simulink model "WorkingModel"  (R2020b)
settings: Solver=VariableStepAuto  StartTime=0.0  StopTime=10.0  RelTol=1e-3
model workspace: external: MATLAB File C:\Users\camka\Documents\Code\MATLAB\RiBBIT\Simscape Hexacopter Model\Model_DataFile1.m (data not in the file)
values from neighbouring files (symbols this model uses):
  D = 12    [Startup.m]
  P = 3.8    [Startup.m]
  X = [ 0, 0, 5, 5, 5, 5, 0]*1    [Path_Construction_Demo_Script.m]
  Y = [ 0, 0, 0, 0, 5, 5, 5]*1    [Path_Construction_Demo_Script.m]
  Z = [ 1, 1, 1, 1, 1, 1, 1]*0    [Path_Construction_Demo_Script.m]
undefined symbols (not defined in the file or in its folder): smiData
libraries: sm_lib x705, fl_lib x72, nesl_utility x16
(part 1 of 12)
settings Model: Creator=camka  LastModifiedBy=camka

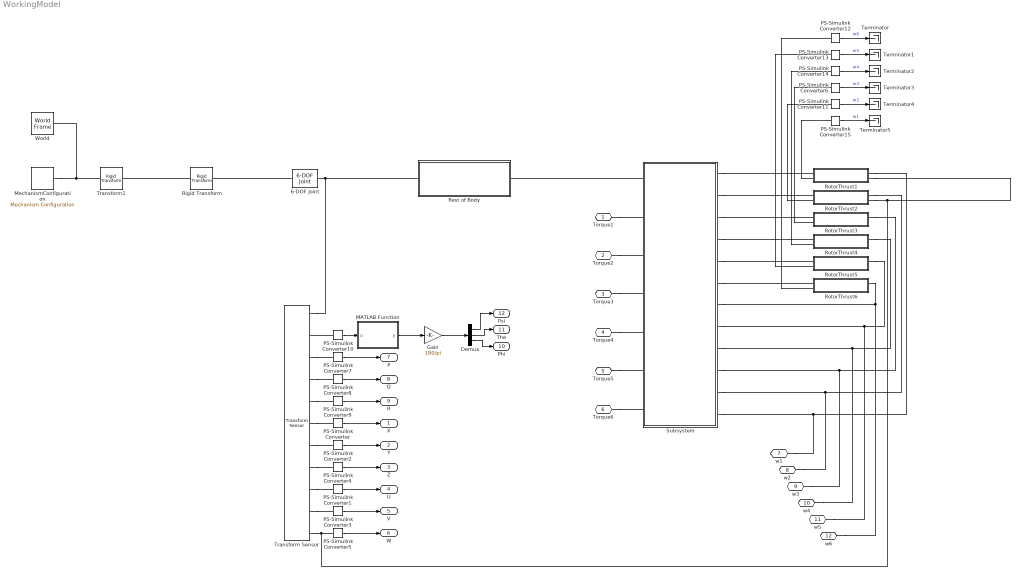
== system WorkingModel ==
  6-DOF Joint : sm_lib/Joints/6-DOF Joint  JointMode=Normal  SenseConstraintForce=off  SenseConstraintForceX=off  SenseConstraintForceY=off  SenseConstraintForceZ=off  SenseConstraintTorque=off  SenseConstraintTorqueX=off  SenseConstraintTorqueY=off  SenseConstraintTorqueZ=off  SenseTotalForce=off  SenseTotalForceX=off  SenseTotalForceY=off  SenseTotalForceZ=off  SenseTotalTorque=off  SenseTotalTorqueX=off  SenseTotalTorqueY=off  SenseTotalTorqueZ=off  CompositeWrenchDir=FollowerOnBase  CompositeWrenchFrame=BaseFrame  PxEquilibriumPosition=0  PxEquilibriumPositionUnits=m  PxSpringStiffness=0  PxSpringStiffnessUnits=N/m  PxDampingCoefficient=0  PxDampingCoefficientUnits=N/(m/s)  PxTorqueActuationMode=NoTorque  PxMotionActuationMode=ComputedMotion  PxSensePosition=off  PxSenseVelocity=off  PxSenseAcceleration=off  PxSenseTorqueForce=off  PxSenseLowerLimitTorqueForce=off  PxSenseUpperLimitTorqueForce=off  PxLowerLimitSpecify=off  PxLowerLimitBound=-1  PxLowerLimitBoundUnits=m  PxLowerLimitStiffness=1e6  PxLowerLimitStiffnessUnits=N/m  PxLowerLimitDamping=1e3  PxLowerLimitDampingUnits=N/(m/s)  PxLowerLimitTransitionRegionWidth=1e-4  PxLowerLimitTransitionRegionWidthUnits=m  PxUpperLimitSpecify=off  PxUpperLimitBound=1  PxUpperLimitBoundUnits=m  PxUpperLimitStiffness=1e6  PxUpperLimitStiffnessUnits=N/m  PxUpperLimitDamping=1e3  PxUpperLimitDampingUnits=N/(m/s)  PxUpperLimitTransitionRegionWidth=1e-4  PxUpperLimitTransitionRegionWidthUnits=m  PxPositionTargetSpecify=off  PxPositionTargetPriority=High  PxPositionTargetValue=0  PxPositionTargetValueUnits=m  PxVelocityTargetSpecify=off  PxVelocityTargetPriority=High  PxVelocityTargetValue=0  PxVelocityTargetValueUnits=m/s  PyEquilibriumPosition=0  PyEquilibriumPositionUnits=m  PySpringStiffness=0  PySpringStiffnessUnits=N/m  PyDampingCoefficient=0  PyDampingCoefficientUnits=N/(m/s)  PyTorqueActuationMode=NoTorque  PyMotionActuationMode=ComputedMotion  PySensePosition=off  PySenseVelocity=off  PySenseAcceleration=off  PySenseTorqueForce=off  PySenseLowerLimitTorqueForce=off  PySenseUpperLimitTorqueForce=off  PyLowerLimitSpecify=off  PyLowerLimitBound=-1  PyLowerLimitBoundUnits=m  PyLowerLimitStiffness=1e6  PyLowerLimitStiffnessUnits=N/m  PyLowerLimitDamping=1e3  PyLowerLimitDampingUnits=N/(m/s)  PyLowerLimitTransitionRegionWidth=1e-4  PyLowerLimitTransitionRegionWidthUnits=m  PyUpperLimitSpecify=off  PyUpperLimitBound=1  PyUpperLimitBoundUnits=m  PyUpperLimitStiffness=1e6  PyUpperLimitStiffnessUnits=N/m  PyUpperLimitDamping=1e3  PyUpperLimitDampingUnits=N/(m/s)  PyUpperLimitTransitionRegionWidth=1e-4  PyUpperLimitTransitionRegionWidthUnits=m  PyPositionTargetSpecify=off  PyPositionTargetPriority=High  PyPositionTargetValue=0  PyPositionTargetValueUnits=m  PyVelocityTargetSpecify=off  PyVelocityTargetPriority=High  PyVelocityTargetValue=0  PyVelocityTargetValueUnits=m/s  PzEquilibriumPosition=0  PzEquilibriumPositionUnits=m  PzSpringStiffness=0  PzSpringStiffnessUnits=N/m  PzDampingCoefficient=0  PzDampingCoefficientUnits=N/(m/s)  PzTorqueActuationMode=NoTorque  PzMotionActuationMode=ComputedMotion  PzSensePosition=off  PzSenseVelocity=off  PzSenseAcceleration=off  PzSenseTorqueForce=off  PzSenseLowerLimitTorqueForce=off  PzSenseUpperLimitTorqueForce=off  PzLowerLimitSpecify=off  PzLowerLimitBound=-1  PzLowerLimitBoundUnits=m  PzLowerLimitStiffness=1e6  PzLowerLimitStiffnessUnits=N/m  PzLowerLimitDamping=1e3  PzLowerLimitDampingUnits=N/(m/s)  PzLowerLimitTransitionRegionWidth=1e-4  PzLowerLimitTransitionRegionWidthUnits=m  PzUpperLimitSpecify=off  PzUpperLimitBound=1  PzUpperLimitBoundUnits=m  PzUpperLimitStiffness=1e6  PzUpperLimitStiffnessUnits=N/m  PzUpperLimitDamping=1e3  PzUpperLimitDampingUnits=N/(m/s)  PzUpperLimitTransitionRegionWidth=1e-4  PzUpperLimitTransitionRegionWidthUnits=m  PzPositionTargetSpecify=off  PzPositionTargetPriority=High  PzPositionTargetValue=-1  PzPositionTargetValueUnits=m  PzVelocityTargetSpecify=off  PzVelocityTargetPriority=High  PzVelocityTargetValue=0  PzVelocityTargetValueUnits=m/s  SphDefPosRotationMethod=None  SphDefPosRotationAngleUnits=deg  SphDefPosRotationStandardAxis=+Z  SphDefPosRotationAngle=0  SphDefPosRotationArbitraryAxis=[0 0 1]  SphDefPosFollAlignAxisA=+X  SphDefPosBaseAlignAxisA=+Y  SphDefPosFollAlignAxisB=+Y  SphDefPosBaseAlignAxisB=+Z  SphDefPosRotationSequenceAxes=FollowerAxes  SphDefPosRotationSequence=XYX  SphDefPosRotationSequenceAngles=[0 0 0]  SphDefPosRotationSequenceAnglesUnits=deg  SphDefPosRotationMatrix=[1 0 0; 0 1 0; 0 0 1]  SphEqPosRotationMethod=None  SphEqPosRotationAngleUnits=deg  SphEqPosRotationStandardAxis=+Z  SphEqPosRotationAngle=0  SphEqPosRotationArbitraryAxis=[0 0 1]  SphEqPosFollAlignAxisA=+X  SphEqPosBaseAlignAxisA=+Y  SphEqPosFollAlignAxisB=+Y  SphEqPosBaseAlignAxisB=+Z  SphEqPosRotationSequenceAxes=FollowerAxes  SphEqPosRotationSequence=XYX  SphEqPosRotationSequenceAngles=[0 0 0]  SphEqPosRotationSequenceAnglesUnits=deg  SphEqPosRotationMatrix=[1 0 0; 0 1 0; 0 0 1]  SphSpringStiffness=0  SphSpringStiffnessUnits=N*m/deg  SphDampingCoefficient=0  SphDampingCoefficientUnits=N*m/(deg/s)  SphActuateTorqueX=off  SphActuateTorqueY=off  SphActuateTorqueZ=off  SphActuateTorque=off  SphTorqueActuationMode=NoTorque  SphMotionActuationMode=ComputedMotion  SphActuationFrame=BaseFrame  SphSensePosition=off  SphSenseVelocityX=off  SphSenseVelocityY=off  SphSenseVelocityZ=off  SphSenseVelocity=off  SphSenseAccelerationX=off  SphSenseAccelerationY=off  SphSenseAccelerationZ=off  SphSenseAcceleration=off  SphSenseTorqueX=off  SphSenseTorqueY=off  SphSenseTorqueZ=off  SphSenseTorqueForce=off  SphSenseLowerLimitTorqueMag=off  SphSenseUpperLimitTorqueMag=off  SphSensingFrame=BaseFrame  SphLowerLimitSpecify=off  SphLowerLimitBound=15  SphLowerLimitBoundUnits=deg  SphLowerLimitStiffness=1e4  SphLowerLimitStiffnessUnits=N*m/deg  SphLowerLimitDamping=10  SphLowerLimitDampingUnits=N*m/(deg/s)  SphLowerLimitTransitionRegionWidth=0.1  SphLowerLimitTransitionRegionWidthUnits=deg  SphUpperLimitSpecify=off  SphUpperLimitBound=45  SphUpperLimitBoundUnits=deg  SphUpperLimitStiffness=1e4  SphUpperLimitStiffnessUnits=N*m/deg  SphUpperLimitDamping=10  SphUpperLimitDampingUnits=N*m/(deg/s)  SphUpperLimitTransitionRegionWidth=0.1  SphUpperLimitTransitionRegionWidthUnits=deg  SphPositionTargetRotationMethod=None  SphPositionTargetRotationAngleUnits=deg  SphPositionTargetRotationStandardAxis=+Z  SphPositionTargetRotationAngle=0  SphPositionTargetRotationArbitraryAxis=[0 0 1]  SphPositionTargetFollAlignAxisA=+X  SphPositionTargetBaseAlignAxisA=+Y  SphPositionTargetFollAlignAxisB=+Y  SphPositionTargetBaseAlignAxisB=+Z  SphPositionTargetRotationSequenceAxes=FollowerAxes  SphPositionTargetRotationSequence=XYX  SphPositionTargetRotationSequenceAngles=[0 0 0]  SphPositionTargetRotationSequenceAnglesUnits=deg  SphPositionTargetRotationMatrix=[1 0 0; 0 1 0; 0 0 1]  SphPositionTargetSpecify=off  SphPositionTargetPriority=High  SphVelocityTargetValue=[0 0 0]  SphVelocityTargetValueUnits=deg/s  SphVelocityTargetSpecify=off  SphVelocityTargetPriority=High  SphVelocityTargetInFollowerFrame=on
  Demux : Demux  Outputs=3
  Gain : Gain  Gain=180/pi
  MATLAB Function : MATLAB Function  TreatAsAtomicUnit=on
  MechanismConfiguration : sm_lib/Utilities/Mechanism Configuration  UniformGravity=Constant  GravityVector=[0 0 0]  GravityVectorUnits=m/s^2  GravityUnits=m/s^2  LinearizationDelta=0.001  JointModeTransitionNonlinearIterations=2
  PS-Simulink Converter{,1..15} (16 alike) : nesl_utility/PS-Simulink Converter  PhysicalDomain=network_engine_domain  SubClassName=ps_output  LeftPortType=input  RightPortType=output  PseudoPeriodic=off  Frequencies=[]  Unit=inherit  AffineConversion=off
  Rest of Body : Subsystem
  Rigid Transform : sm_lib/Frames and Transforms/Rigid Transform  TranslationMethod=None  TranslationStandardOffset=0  TranslationLengthUnit=m  TranslationStandardAxis=+Z  TranslationCartesianOffset=[0 0 0]  TranslationROffset=0  TranslationROffsetUnits=m  TranslationZOffset=0  TranslationZOffsetUnits=m  TranslationThetaOffset=0  TranslationThetaOffsetUnits=deg  RotationMethod=RotationSequence  RotationAngleUnits=deg  RotationStandardAxis=+Z  RotationAngle=0.0  RotationArbitraryAxis=[0 0 1]  FollAlignAxisA=+X  BaseAlignAxisA=+Y  FollAlignAxisB=+Y  BaseAlignAxisB=+Z  RotationSequenceAxes=BaseAxes  RotationSequence=XZX  RotationSequenceAngles=[-90 90 0]  RotationSequenceAnglesUnits=deg  RotationMatrix=[1 0 0; 0 1 0; 0 0 1]
  RotorThrust1 : Subsystem
  RotorThrust2 : Subsystem
  RotorThrust3 : Subsystem
  RotorThrust4 : Subsystem
  RotorThrust5 : Subsystem
  RotorThrust6 : Subsystem
  Subsystem : Subsystem
  Terminator{,1..5} (6 alike) : Terminator
  Transform Sensor : sm_lib/Frames and Transforms/Transform Sensor  MeasurementFrame=NonRotatingBase  SenseAngle=off  SenseAxis=off  SenseAngle1=off  SenseAngle2=off  SenseAngle3=off  SenseQ=on  SenseR=off  SenseOmegaX=on  SenseOmegaY=on  SenseOmegaZ=on  SenseOmega1=off  SenseOmega2=off  SenseOmega3=off  SenseQDot=off  SenseRDot=off  SenseAlphaX=off  SenseAlphaY=off  SenseAlphaZ=off  SenseAlpha1=off  SenseAlpha2=off  SenseAlpha3=off  SenseQDDot=off  SenseRDDot=off  SenseX=on  SenseY=on  SenseZ=on  SenseRad=off  SenseAzim=off  SenseDist=off  SenseInc=off  SenseXDot=on  SenseYDot=on  SenseZDot=on  SenseRadDot=off  SenseAzimDot=off  SenseDistDot=off  SenseIncDot=off  SenseXDDot=off  SenseYDDot=off  SenseZDDot=off  SenseRadDDot=off  SenseAzimDDot=off  SenseDistDDot=off  SenseIncDDot=off
  Transform1 : sm_lib/Frames and Transforms/Rigid Transform  TranslationMethod=Cartesian  TranslationStandardOffset=0  TranslationLengthUnit=cm  TranslationStandardAxis=+Z  TranslationCartesianOffset=smiData.RigidTransform(6).translation  TranslationROffset=0  TranslationROffsetUnits=m  TranslationZOffset=0  TranslationZOffsetUnits=m  TranslationThetaOffset=0  TranslationThetaOffsetUnits=deg  RotationMethod=ArbitraryAxis  RotationAngleUnits=rad  RotationStandardAxis=+Z  RotationAngle=smiData.RigidTransform(6).angle  RotationArbitraryAxis=smiData.RigidTransform(6).axis  FollAlignAxisA=+X  BaseAlignAxisA=+Y  FollAlignAxisB=+Y  BaseAlignAxisB=+Z  RotationSequenceAxes=FollowerAxes  RotationSequence=XYX  RotationSequenceAngles=[0 0 0]  RotationSequenceAnglesUnits=deg  RotationMatrix=[1 0 0; 0 1 0; 0 0 1]
  World : sm_lib/Frames and Transforms/World Frame
  Torque1 : PMIOPort  Side=Left
  Torque2 : PMIOPort  Port=2  Side=Left
  Torque3 : PMIOPort  Port=3  Side=Left
  Torque4 : PMIOPort  Port=4  Side=Left
  Torque5 : PMIOPort  Port=5  Side=Left
  Torque6 : PMIOPort  Port=6  Side=Left
  w1 : PMIOPort  Port=7  Side=Left
  w2 : PMIOPort  Port=8  Side=Left
  w3 : PMIOPort  Port=9  Side=Left
  w4 : PMIOPort  Port=10  Side=Left
  w5 : PMIOPort  Port=11  Side=Left
  w6 : PMIOPort  Port=12  Side=Left
  X : Outport
  Y : Outport  Port=2
  Z : Outport  Port=3
  U : Outport  Port=4
  V : Outport  Port=5
  W : Outport  Port=6
  P : Outport  Port=7
  Q : Outport  Port=8
  R : Outport  Port=9
  Phi : Outport  Port=10
  The : Outport  Port=11
  Psi : Outport  Port=12
  wires:
  Demux/2 -> The/1
  PS-Simulink Converter10/1 -> MATLAB Function/1(u)
  MATLAB Function/1(y) -> Gain/1
  PS-Simulink Converter1/1 -> U/1
  PS-Simulink Converter/1 -> X/1
  Demux/3 -> Phi/1
  PS-Simulink Converter4/1 -> Z/1
  PS-Simulink Converter3/1 -> V/1
  Demux/1 -> Psi/1
  PS-Simulink Converter7/1 -> P/1
  PS-Simulink Converter5/1 -> W/1
  PS-Simulink Converter8/1 -> Q/1
  PS-Simulink Converter2/1 -> Y/1
  PS-Simulink Converter9/1 -> R/1
  Gain/1 -> Demux/1
  PS-Simulink Converter13/1 -> Terminator1/1  "w5"
  PS-Simulink Converter14/1 -> Terminator2/1  "w4"
  PS-Simulink Converter12/1 -> Terminator/1  "w6"
  PS-Simulink Converter6/1 -> Terminator3/1  "w3"
  PS-Simulink Converter11/1 -> Terminator4/1  "w2"
  PS-Simulink Converter15/1 -> Terminator5/1  "w1"
  connections:
  World/RConn1 -- MechanismConfiguration/RConn1 -- Transform1/LConn1
  Rigid Transform/LConn1 -- Transform1/RConn1
  RotorThrust2/LConn2 -- RotorThrust1/LConn2 -- Transform Sensor/RConn11 -- PS-Simulink Converter5/LConn1
  Transform Sensor/RConn4 -- PS-Simulink Converter8/LConn1
  Transform Sensor/RConn9 -- PS-Simulink Converter1/LConn1
  Transform Sensor/RConn7 -- PS-Simulink Converter2/LConn1
  Transform Sensor/RConn8 -- PS-Simulink Converter4/LConn1
  6-DOF Joint/RConn1 -- Rest of Body/RConn1 -- Transform Sensor/RConn1
  Transform Sensor/RConn6 -- PS-Simulink Converter/LConn1
  Transform Sensor/RConn3 -- PS-Simulink Converter7/LConn1
  6-DOF Joint/LConn1 -- Rigid Transform/RConn1
  Transform Sensor/RConn10 -- PS-Simulink Converter3/LConn1
  Transform Sensor/RConn5 -- PS-Simulink Converter9/LConn1
  PS-Simulink Converter10/LConn1 -- Transform Sensor/RConn2
  Subsystem/LConn1 -- Rest of Body/LConn1
  RotorThrust4/LConn1 -- Subsystem/RConn9 -- w4/RConn1
  RotorThrust3/LConn1 -- Subsystem/RConn10 -- w3/RConn1
  RotorThrust2/LConn1 -- Subsystem/RConn11 -- w2/RConn1
  RotorThrust6/LConn1 -- Subsystem/RConn7 -- w6/RConn1
  RotorThrust5/LConn1 -- Subsystem/RConn8 -- w5/RConn1
  RotorThrust1/LConn1 -- Subsystem/RConn12 -- w1/RConn1
  PS-Simulink Converter12/LConn1 -- RotorThrust6/RConn2
  Subsystem/RConn6 -- RotorThrust6/RConn1
  Subsystem/RConn2 -- RotorThrust2/RConn1
  PS-Simulink Converter11/LConn1 -- RotorThrust2/RConn2
  PS-Simulink Converter6/LConn1 -- RotorThrust3/RConn2
  PS-Simulink Converter15/LConn1 -- RotorThrust1/RConn2
  PS-Simulink Converter13/LConn1 -- RotorThrust5/RConn2
  PS-Simulink Converter14/LConn1 -- RotorThrust4/RConn2
  Subsystem/RConn5 -- RotorThrust5/RConn1
  Subsystem/RConn3 -- RotorThrust3/RConn1
  Subsystem/RConn4 -- RotorThrust4/RConn1
  Subsystem/RConn1 -- RotorThrust1/RConn1
  Torque1/RConn1 -- Subsystem/LConn2
  Torque2/RConn1 -- Subsystem/LConn3
  Torque3/RConn1 -- Subsystem/LConn4
  Torque4/RConn1 -- Subsystem/LConn5
  Torque5/RConn1 -- Subsystem/LConn6
  Torque6/RConn1 -- Subsystem/LConn7

== system WorkingModel/Rest of Body ==
  ReferenceFrame : sm_lib/Frames and Transforms/Reference Frame
  ReferenceFrame1 : sm_lib/Frames and Transforms/Reference Frame
  ReferenceFrame2 : sm_lib/Frames and Transforms/Reference Frame
  Subsystem : Subsystem
  Subsystem1 : Subsystem
  Transform1 : sm_lib/Frames and Transforms/Rigid Transform  TranslationMethod=Cartesian  TranslationStandardOffset=0  TranslationLengthUnit=cm  TranslationStandardAxis=+Z  TranslationCartesianOffset=smiData.RigidTransform(5).translation  TranslationROffset=0  TranslationROffsetUnits=m  TranslationZOffset=0  TranslationZOffsetUnits=m  TranslationThetaOffset=0  TranslationThetaOffsetUnits=deg  RotationMethod=ArbitraryAxis  RotationAngleUnits=rad  RotationStandardAxis=+Z  RotationAngle=smiData.RigidTransform(5).angle  RotationArbitraryAxis=smiData.RigidTransform(5).axis  FollAlignAxisA=+X  BaseAlignAxisA=+Y  FollAlignAxisB=+Y  BaseAlignAxisB=+Z  RotationSequenceAxes=FollowerAxes  RotationSequence=XYX  RotationSequenceAngles=[0 0 0]  RotationSequenceAnglesUnits=deg  RotationMatrix=[1 0 0; 0 1 0; 0 0 1]
  Transform34 : sm_lib/Frames and Transforms/Rigid Transform  TranslationMethod=Cartesian  TranslationStandardOffset=0  TranslationLengthUnit=cm  TranslationStandardAxis=+Z  TranslationCartesianOffset=smiData.RigidTransform(128).translation  TranslationROffset=0  TranslationROffsetUnits=m  TranslationZOffset=0  TranslationZOffsetUnits=m  TranslationThetaOffset=0  TranslationThetaOffsetUnits=deg  RotationMethod=ArbitraryAxis  RotationAngleUnits=rad  RotationStandardAxis=+Z  RotationAngle=smiData.RigidTransform(128).angle  RotationArbitraryAxis=smiData.RigidTransform(128).axis  FollAlignAxisA=+X  BaseAlignAxisA=+Y  FollAlignAxisB=+Y  BaseAlignAxisB=+Z  RotationSequenceAxes=FollowerAxes  RotationSequence=XYX  RotationSequenceAngles=[0 0 0]  RotationSequenceAnglesUnits=deg  RotationMatrix=[1 0 0; 0 1 0; 0 0 1]
  Transform5 : sm_lib/Frames and Transforms/Rigid Transform  TranslationMethod=Cartesian  TranslationStandardOffset=0  TranslationLengthUnit=cm  TranslationStandardAxis=+Z  TranslationCartesianOffset=smiData.RigidTransform(236).translation  TranslationROffset=0  TranslationROffsetUnits=m  TranslationZOffset=0  TranslationZOffsetUnits=m  TranslationThetaOffset=0  TranslationThetaOffsetUnits=deg  RotationMethod=ArbitraryAxis  RotationAngleUnits=rad  RotationStandardAxis=+Z  RotationAngle=smiData.RigidTransform(236).angle  RotationArbitraryAxis=smiData.RigidTransform(236).axis  FollAlignAxisA=+X  BaseAlignAxisA=+Y  FollAlignAxisB=+Y  BaseAlignAxisB=+Z  RotationSequenceAxes=FollowerAxes  RotationSequence=XYX  RotationSequenceAngles=[0 0 0]  RotationSequenceAnglesUnits=deg  RotationMatrix=[1 0 0; 0 1 0; 0 0 1]
  Transform2 : PMIOPort  Side=Right
  Transform3 : PMIOPort  Port=2  Side=Left
  connections:
  Transform1/LConn1 -- Transform5/LConn1 -- ReferenceFrame/RConn1
  ReferenceFrame1/RConn1 -- Transform3/RConn1 -- Transform34/RConn1 -- Subsystem1/LConn1
  ReferenceFrame2/RConn1 -- Transform34/LConn1 -- Subsystem/LConn1 -- Transform5/RConn1
  Transform1/RConn1 -- Transform2/RConn1

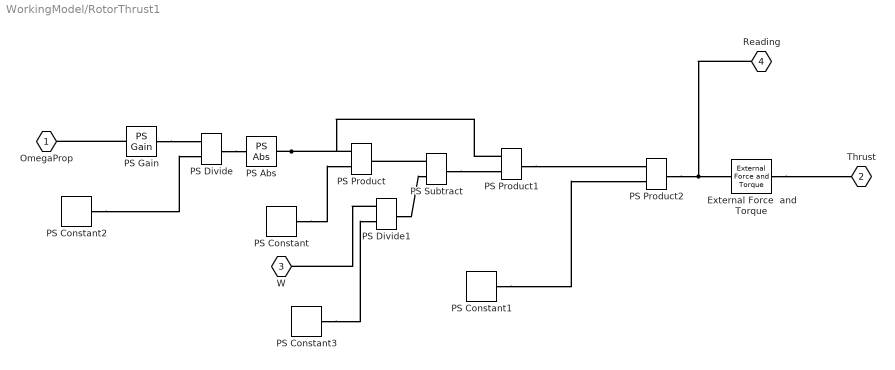
== system WorkingModel/RotorThrust1 ==
  External Force  and Torque : sm_lib/Forces and Torques/External Force and Torque  ForceResolutionFrame=AttachedFrame  EnableForceX=off  EnableForceY=off  EnableForceZ=on  EnableForce=off  TorqueResolutionFrame=AttachedFrame  EnableTorqueX=off  EnableTorqueY=off  EnableTorqueZ=off  EnableTorque=off
  PS Abs : fl_lib/Physical Signals/Nonlinear Operators/PS Abs
      settings: SourceProductBaseCode=SS  InternalSimscapePortConfiguration="{\"Bottom\":[],\"Left\":[{\"id\":\"I\",\"label\":\"\",\"type\":\"input\"}],\"Right\":[{\"id\":\"O\",\"label\":\"\",\"type\":\"output\"}],\"Top\":[]}"
  PS Constant : fl_lib/Physical Signals/Sources/PS Constant  constant=4.23333e-4*P
  PS Constant1 : fl_lib/Physical Signals/Sources/PS Constant  constant=4.392399e-8*D^3.5/sqrt(P) N
  PS Constant2 : fl_lib/Physical Signals/Sources/PS Constant  constant=1 rad/s
  PS Constant3 : fl_lib/Physical Signals/Sources/PS Constant  constant=1 m/s
  PS Divide : fl_lib/Physical Signals/Functions/PS Divide
      settings: SourceProductBaseCode=SS
  PS Divide1 : fl_lib/Physical Signals/Functions/PS Divide
      settings: SourceProductBaseCode=SS
  PS Gain : fl_lib/Physical Signals/Functions/PS Gain  gain=30/pi
  PS Product : fl_lib/Physical Signals/Functions/PS Product
  PS Product1 : fl_lib/Physical Signals/Functions/PS Product
  PS Product2 : fl_lib/Physical Signals/Functions/PS Product
  PS Subtract : fl_lib/Physical Signals/Functions/PS Subtract
  OmegaProp : PMIOPort  Side=Left
  Thrust : PMIOPort  Port=2  Side=Right
  W : PMIOPort  Port=3  Side=Left
  Reading : PMIOPort  Port=4  Side=Right
  connections:
  External Force  and Torque/RConn1 -- Thrust/RConn1
  PS Product2/RConn1 -- Reading/RConn1 -- External Force  and Torque/LConn1
  PS Gain/LConn1 -- OmegaProp/RConn1
  PS Constant/RConn1 -- PS Product/LConn2
  PS Abs/RConn1 -- PS Product/LConn1 -- PS Product1/LConn1
  PS Subtract/LConn1 -- PS Product/RConn1
  PS Divide1/LConn1 -- W/RConn1
  PS Subtract/RConn1 -- PS Product1/LConn2
  PS Constant1/RConn1 -- PS Product2/LConn2
  PS Product1/RConn1 -- PS Product2/LConn1
  PS Gain/RConn1 -- PS Divide/LConn1
  PS Divide/RConn1 -- PS Abs/LConn1
  PS Constant2/RConn1 -- PS Divide/LConn2
  PS Divide1/RConn1 -- PS Subtract/LConn2
  PS Constant3/RConn1 -- PS Divide1/LConn2

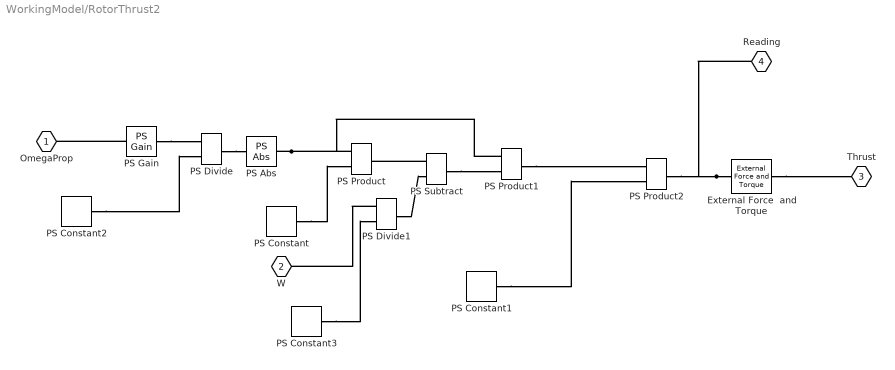
== system WorkingModel/RotorThrust2 ==
  External Force  and Torque : sm_lib/Forces and Torques/External Force and Torque  ForceResolutionFrame=AttachedFrame  EnableForceX=off  EnableForceY=off  EnableForceZ=on  EnableForce=off  TorqueResolutionFrame=AttachedFrame  EnableTorqueX=off  EnableTorqueY=off  EnableTorqueZ=off  EnableTorque=off
  PS Abs : fl_lib/Physical Signals/Nonlinear Operators/PS Abs
      settings: SourceProductBaseCode=SS  InternalSimscapePortConfiguration="{\"Bottom\":[],\"Left\":[{\"id\":\"I\",\"label\":\"\",\"type\":\"input\"}],\"Right\":[{\"id\":\"O\",\"label\":\"\",\"type\":\"output\"}],\"Top\":[]}"
  PS Constant : fl_lib/Physical Signals/Sources/PS Constant  constant=4.23333e-4*P
  PS Constant1 : fl_lib/Physical Signals/Sources/PS Constant  constant=4.392399e-8*D^3.5/sqrt(P) N
  PS Constant2 : fl_lib/Physical Signals/Sources/PS Constant  constant=1 rad/s
  PS Constant3 : fl_lib/Physical Signals/Sources/PS Constant  constant=1 m/s
  PS Divide : fl_lib/Physical Signals/Functions/PS Divide
      settings: SourceProductBaseCode=SS
  PS Divide1 : fl_lib/Physical Signals/Functions/PS Divide
      settings: SourceProductBaseCode=SS
  PS Gain : fl_lib/Physical Signals/Functions/PS Gain  gain=30/pi
  PS Product : fl_lib/Physical Signals/Functions/PS Product
  PS Product1 : fl_lib/Physical Signals/Functions/PS Product
  PS Product2 : fl_lib/Physical Signals/Functions/PS Product
  PS Subtract : fl_lib/Physical Signals/Functions/PS Subtract
  OmegaProp : PMIOPort  Side=Left
  W : PMIOPort  Port=2  Side=Left
  Thrust : PMIOPort  Port=3  Side=Right
  Reading : PMIOPort  Port=4  Side=Right
  connections:
  External Force  and Torque/RConn1 -- Thrust/RConn1
  External Force  and Torque/LConn1 -- PS Product2/RConn1 -- Reading/RConn1
  PS Gain/LConn1 -- OmegaProp/RConn1
  PS Constant/RConn1 -- PS Product/LConn2
  PS Abs/RConn1 -- PS Product/LConn1 -- PS Product1/LConn1
  PS Subtract/LConn1 -- PS Product/RConn1
  PS Divide1/LConn1 -- W/RConn1
  PS Subtract/RConn1 -- PS Product1/LConn2
  PS Constant1/RConn1 -- PS Product2/LConn2
  PS Product1/RConn1 -- PS Product2/LConn1
  PS Gain/RConn1 -- PS Divide/LConn1
  PS Divide/RConn1 -- PS Abs/LConn1
  PS Constant2/RConn1 -- PS Divide/LConn2
  PS Divide1/RConn1 -- PS Subtract/LConn2
  PS Constant3/RConn1 -- PS Divide1/LConn2

== system WorkingModel/RotorThrust3 ==
  External Force  and Torque : sm_lib/Forces and Torques/External Force and Torque  ForceResolutionFrame=AttachedFrame  EnableForceX=off  EnableForceY=off  EnableForceZ=on  EnableForce=off  TorqueResolutionFrame=AttachedFrame  EnableTorqueX=off  EnableTorqueY=off  EnableTorqueZ=off  EnableTorque=off
  PS Abs : fl_lib/Physical Signals/Nonlinear Operators/PS Abs
      settings: SourceProductBaseCode=SS  InternalSimscapePortConfiguration="{\"Bottom\":[],\"Left\":[{\"id\":\"I\",\"label\":\"\",\"type\":\"input\"}],\"Right\":[{\"id\":\"O\",\"label\":\"\",\"type\":\"output\"}],\"Top\":[]}"
  PS Constant : fl_lib/Physical Signals/Sources/PS Constant  constant=4.23333e-4*P
  PS Constant1 : fl_lib/Physical Signals/Sources/PS Constant  constant=4.392399e-8*D^3.5/sqrt(P) N
  PS Constant2 : fl_lib/Physical Signals/Sources/PS Constant  constant=1 rad/s
  PS Constant3 : fl_lib/Physical Signals/Sources/PS Constant  constant=1 m/s
  PS Divide : fl_lib/Physical Signals/Functions/PS Divide
      settings: SourceProductBaseCode=SS
  PS Divide1 : fl_lib/Physical Signals/Functions/PS Divide
      settings: SourceProductBaseCode=SS
  PS Gain : fl_lib/Physical Signals/Functions/PS Gain  gain=30/pi
  PS Product : fl_lib/Physical Signals/Functions/PS Product
  PS Product1 : fl_lib/Physical Signals/Functions/PS Product
  PS Product2 : fl_lib/Physical Signals/Functions/PS Product
  PS Subtract : fl_lib/Physical Signals/Functions/PS Subtract
  OmegaProp : PMIOPort  Side=Left
  Thrust : PMIOPort  Port=2  Side=Right
  W : PMIOPort  Port=3  Side=Left
  Reading : PMIOPort  Port=4  Side=Right
  connections:
  External Force  and Torque/RConn1 -- Thrust/RConn1
  External Force  and Torque/LConn1 -- PS Product2/RConn1 -- Reading/RConn1
  PS Gain/LConn1 -- OmegaProp/RConn1
  PS Constant/RConn1 -- PS Product/LConn2
  PS Abs/RConn1 -- PS Product/LConn1 -- PS Product1/LConn1
  PS Subtract/LConn1 -- PS Product/RConn1
  PS Divide1/LConn1 -- W/RConn1
  PS Subtract/RConn1 -- PS Product1/LConn2
  PS Constant1/RConn1 -- PS Product2/LConn2
  PS Product1/RConn1 -- PS Product2/LConn1
  PS Gain/RConn1 -- PS Divide/LConn1
  PS Divide/RConn1 -- PS Abs/LConn1
  PS Constant2/RConn1 -- PS Divide/LConn2
  PS Divide1/RConn1 -- PS Subtract/LConn2
  PS Constant3/RConn1 -- PS Divide1/LConn2

== system WorkingModel/RotorThrust4 ==
  External Force  and Torque : sm_lib/Forces and Torques/External Force and Torque  ForceResolutionFrame=AttachedFrame  EnableForceX=off  EnableForceY=off  EnableForceZ=on  EnableForce=off  TorqueResolutionFrame=AttachedFrame  EnableTorqueX=off  EnableTorqueY=off  EnableTorqueZ=off  EnableTorque=off
  PS Abs : fl_lib/Physical Signals/Nonlinear Operators/PS Abs
      settings: SourceProductBaseCode=SS  InternalSimscapePortConfiguration="{\"Bottom\":[],\"Left\":[{\"id\":\"I\",\"label\":\"\",\"type\":\"input\"}],\"Right\":[{\"id\":\"O\",\"label\":\"\",\"type\":\"output\"}],\"Top\":[]}"
  PS Constant : fl_lib/Physical Signals/Sources/PS Constant  constant=4.23333e-4*P
  PS Constant1 : fl_lib/Physical Signals/Sources/PS Constant  constant=4.392399e-8*D^3.5/sqrt(P) N
  PS Constant2 : fl_lib/Physical Signals/Sources/PS Constant  constant=1 rad/s
  PS Constant3 : fl_lib/Physical Signals/Sources/PS Constant  constant=1 m/s
  PS Divide : fl_lib/Physical Signals/Functions/PS Divide
      settings: SourceProductBaseCode=SS
  PS Divide1 : fl_lib/Physical Signals/Functions/PS Divide
      settings: SourceProductBaseCode=SS
  PS Gain : fl_lib/Physical Signals/Functions/PS Gain  gain=30/pi
  PS Product : fl_lib/Physical Signals/Functions/PS Product
  PS Product1 : fl_lib/Physical Signals/Functions/PS Product
  PS Product2 : fl_lib/Physical Signals/Functions/PS Product
  PS Subtract : fl_lib/Physical Signals/Functions/PS Subtract
  OmegaProp : PMIOPort  Side=Left
  Thrust : PMIOPort  Port=2  Side=Right
  W : PMIOPort  Port=3  Side=Left
  Reading : PMIOPort  Port=4  Side=Right
  connections:
  External Force  and Torque/RConn1 -- Thrust/RConn1
  External Force  and Torque/LConn1 -- PS Product2/RConn1 -- Reading/RConn1
  PS Gain/LConn1 -- OmegaProp/RConn1
  PS Constant/RConn1 -- PS Product/LConn2
  PS Abs/RConn1 -- PS Product/LConn1 -- PS Product1/LConn1
  PS Subtract/LConn1 -- PS Product/RConn1
  PS Divide1/LConn1 -- W/RConn1
  PS Subtract/RConn1 -- PS Product1/LConn2
  PS Constant1/RConn1 -- PS Product2/LConn2
  PS Product1/RConn1 -- PS Product2/LConn1
  PS Gain/RConn1 -- PS Divide/LConn1
  PS Divide/RConn1 -- PS Abs/LConn1
  PS Constant2/RConn1 -- PS Divide/LConn2
  PS Divide1/RConn1 -- PS Subtract/LConn2
  PS Constant3/RConn1 -- PS Divide1/LConn2

== system WorkingModel/RotorThrust5 ==
  External Force  and Torque : sm_lib/Forces and Torques/External Force and Torque  ForceResolutionFrame=AttachedFrame  EnableForceX=off  EnableForceY=off  EnableForceZ=on  EnableForce=off  TorqueResolutionFrame=AttachedFrame  EnableTorqueX=off  EnableTorqueY=off  EnableTorqueZ=off  EnableTorque=off
  PS Abs : fl_lib/Physical Signals/Nonlinear Operators/PS Abs
      settings: SourceProductBaseCode=SS  InternalSimscapePortConfiguration="{\"Bottom\":[],\"Left\":[{\"id\":\"I\",\"label\":\"\",\"type\":\"input\"}],\"Right\":[{\"id\":\"O\",\"label\":\"\",\"type\":\"output\"}],\"Top\":[]}"
  PS Constant : fl_lib/Physical Signals/Sources/PS Constant  constant=4.23333e-4*P
  PS Constant1 : fl_lib/Physical Signals/Sources/PS Constant  constant=4.392399e-8*D^3.5/sqrt(P) N
  PS Constant2 : fl_lib/Physical Signals/Sources/PS Constant  constant=1 rad/s
  PS Constant3 : fl_lib/Physical Signals/Sources/PS Constant  constant=1 m/s
  PS Divide : fl_lib/Physical Signals/Functions/PS Divide
      settings: SourceProductBaseCode=SS
  PS Divide1 : fl_lib/Physical Signals/Functions/PS Divide
      settings: SourceProductBaseCode=SS
  PS Gain : fl_lib/Physical Signals/Functions/PS Gain  gain=30/pi
  PS Product : fl_lib/Physical Signals/Functions/PS Product
  PS Product1 : fl_lib/Physical Signals/Functions/PS Product
  PS Product2 : fl_lib/Physical Signals/Functions/PS Product
  PS Subtract : fl_lib/Physical Signals/Functions/PS Subtract
  OmegaProp : PMIOPort  Side=Left
  Thrust : PMIOPort  Port=2  Side=Right
  W : PMIOPort  Port=3  Side=Left
  Reading : PMIOPort  Port=4  Side=Right
  connections:
  External Force  and Torque/RConn1 -- Thrust/RConn1
  External Force  and Torque/LConn1 -- PS Product2/RConn1 -- Reading/RConn1
  PS Gain/LConn1 -- OmegaProp/RConn1
  PS Constant/RConn1 -- PS Product/LConn2
  PS Abs/RConn1 -- PS Product/LConn1 -- PS Product1/LConn1
  PS Subtract/LConn1 -- PS Product/RConn1
  PS Divide1/LConn1 -- W/RConn1
  PS Subtract/RConn1 -- PS Product1/LConn2
  PS Constant1/RConn1 -- PS Product2/LConn2
  PS Product1/RConn1 -- PS Product2/LConn1
  PS Gain/RConn1 -- PS Divide/LConn1
  PS Divide/RConn1 -- PS Abs/LConn1
  PS Constant2/RConn1 -- PS Divide/LConn2
  PS Divide1/RConn1 -- PS Subtract/LConn2
  PS Constant3/RConn1 -- PS Divide1/LConn2

== system WorkingModel/RotorThrust6 ==
  External Force  and Torque : sm_lib/Forces and Torques/External Force and Torque  ForceResolutionFrame=AttachedFrame  EnableForceX=off  EnableForceY=off  EnableForceZ=on  EnableForce=off  TorqueResolutionFrame=AttachedFrame  EnableTorqueX=off  EnableTorqueY=off  EnableTorqueZ=off  EnableTorque=off
  PS Abs : fl_lib/Physical Signals/Nonlinear Operators/PS Abs
      settings: SourceProductBaseCode=SS  InternalSimscapePortConfiguration="{\"Bottom\":[],\"Left\":[{\"id\":\"I\",\"label\":\"\",\"type\":\"input\"}],\"Right\":[{\"id\":\"O\",\"label\":\"\",\"type\":\"output\"}],\"Top\":[]}"
  PS Constant : fl_lib/Physical Signals/Sources/PS Constant  constant=4.23333e-4*P
  PS Constant1 : fl_lib/Physical Signals/Sources/PS Constant  constant=4.392399e-8*D^3.5/sqrt(P) N
  PS Constant2 : fl_lib/Physical Signals/Sources/PS Constant  constant=1 rad/s
  PS Constant3 : fl_lib/Physical Signals/Sources/PS Constant  constant=1 m/s
  PS Divide : fl_lib/Physical Signals/Functions/PS Divide
      settings: SourceProductBaseCode=SS
  PS Divide1 : fl_lib/Physical Signals/Functions/PS Divide
      settings: SourceProductBaseCode=SS
  PS Gain : fl_lib/Physical Signals/Functions/PS Gain  gain=30/pi
  PS Product : fl_lib/Physical Signals/Functions/PS Product
  PS Product1 : fl_lib/Physical Signals/Functions/PS Product
  PS Product2 : fl_lib/Physical Signals/Functions/PS Product
  PS Subtract : fl_lib/Physical Signals/Functions/PS Subtract
  OmegaProp : PMIOPort  Side=Left
  Thrust : PMIOPort  Port=2  Side=Right
  W : PMIOPort  Port=3  Side=Left
  Reading : PMIOPort  Port=4  Side=Right
  connections:
  External Force  and Torque/RConn1 -- Thrust/RConn1
  External Force  and Torque/LConn1 -- PS Product2/RConn1 -- Reading/RConn1
  PS Gain/LConn1 -- OmegaProp/RConn1
  PS Constant/RConn1 -- PS Product/LConn2
  PS Abs/RConn1 -- PS Product/LConn1 -- PS Product1/LConn1
  PS Subtract/LConn1 -- PS Product/RConn1
  PS Divide1/LConn1 -- W/RConn1
  PS Subtract/RConn1 -- PS Product1/LConn2
  PS Constant1/RConn1 -- PS Product2/LConn2
  PS Product1/RConn1 -- PS Product2/LConn1
  PS Gain/RConn1 -- PS Divide/LConn1
  PS Divide/RConn1 -- PS Abs/LConn1
  PS Constant2/RConn1 -- PS Divide/LConn2
  PS Divide1/RConn1 -- PS Subtract/LConn2
  PS Constant3/RConn1 -- PS Divide1/LConn2

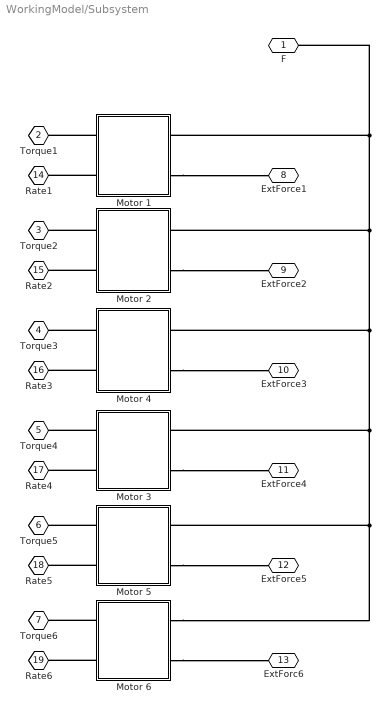
== system WorkingModel/Subsystem ==
  Motor 1 : Subsystem
  Motor 2 : Subsystem
  Motor 3 : Subsystem
  Motor 4 : Subsystem
  Motor 5 : Subsystem
  Motor 6 : Subsystem
  F : PMIOPort  Side=Left
  Torque1 : PMIOPort  Tag=PMCPort  Port=2  Side=Left
  Torque2 : PMIOPort  Tag=PMCPort  Port=3  Side=Left
  Torque3 : PMIOPort  Tag=PMCPort  Port=4  Side=Left
  Torque4 : PMIOPort  Tag=PMCPort  Port=5  Side=Left
  Torque5 : PMIOPort  Tag=PMCPort  Port=6  Side=Left
  Torque6 : PMIOPort  Tag=PMCPort  Port=7  Side=Left
  ExtForce1 : PMIOPort  Port=8  Side=Right
  ExtForce2 : PMIOPort  Port=9  Side=Right
  ExtForce3 : PMIOPort  Port=10  Side=Right
  ExtForce4 : PMIOPort  Port=11  Side=Right
  ExtForce5 : PMIOPort  Port=12  Side=Right
  ExtForc6 : PMIOPort  Port=13  Side=Right
  Rate1 : PMIOPort  Tag=PMCPort  Port=14  Side=Right
  Rate2 : PMIOPort  Tag=PMCPort  Port=15  Side=Right
  Rate3 : PMIOPort  Tag=PMCPort  Port=16  Side=Right
  Rate4 : PMIOPort  Tag=PMCPort  Port=17  Side=Right
  Rate5 : PMIOPort  Tag=PMCPort  Port=18  Side=Right
  Rate6 : PMIOPort  Tag=PMCPort  Port=19  Side=Right
  connections:
  Motor 6/RConn1 -- Motor 5/RConn1 -- Motor 3/RConn1 -- Motor 4/RConn1 -- Motor 2/RConn1 -- Motor 1/RConn1 -- F/RConn1
  Motor 5/LConn2 -- Rate5/RConn1
  Motor 1/LConn2 -- Rate1/RConn1
  Motor 4/LConn2 -- Rate3/RConn1
  Motor 6/LConn2 -- Rate6/RConn1
  Motor 3/LConn1 -- Torque4/RConn1
  Motor 3/LConn2 -- Rate4/RConn1
  Motor 4/LConn1 -- Torque3/RConn1
  Motor 1/LConn1 -- Torque1/RConn1
  Motor 2/LConn1 -- Torque2/RConn1
  Motor 6/LConn1 -- Torque6/RConn1
  Motor 2/LConn2 -- Rate2/RConn1
  Motor 5/LConn1 -- Torque5/RConn1
  Motor 1/RConn2 -- ExtForce1/RConn1
  Motor 6/RConn2 -- ExtForc6/RConn1
  Motor 5/RConn2 -- ExtForce5/RConn1
  Motor 2/RConn2 -- ExtForce2/RConn1
  Motor 4/RConn2 -- ExtForce3/RConn1
  Motor 3/RConn2 -- ExtForce4/RConn1

== system WorkingModel/Rest of Body/Subsystem ==
  DJI_S900_A2_IMU_STEP_1_RIGID : Subsystem
  DJI_S900_GPS_Compass_STEP_1_RIGID : Subsystem
  DJI_S900_GPS_Module_STEP_1_RIGID : Subsystem
  DJI_S900_Landing_Bracket_Attachment_Piece_STEP_1_RIGID : Subsystem
  DJI_S900_Landing_Bracket_Attachment_Piece_STEP_2_RIGID : Subsystem
  DJI_S900_Lower_Assembly_STEP_1_RIGID : Subsystem
  Transform : sm_lib/Frames and Transforms/Rigid Transform  TranslationMethod=Cartesian  TranslationStandardOffset=0  TranslationLengthUnit=cm  TranslationStandardAxis=+Z  TranslationCartesianOffset=smiData.RigidTransform(7).translation  TranslationROffset=0  TranslationROffsetUnits=m  TranslationZOffset=0  TranslationZOffsetUnits=m  TranslationThetaOffset=0  TranslationThetaOffsetUnits=deg  RotationMethod=ArbitraryAxis  RotationAngleUnits=rad  RotationStandardAxis=+Z  RotationAngle=smiData.RigidTransform(7).angle  RotationArbitraryAxis=smiData.RigidTransform(7).axis  FollAlignAxisA=+X  BaseAlignAxisA=+Y  FollAlignAxisB=+Y  BaseAlignAxisB=+Z  RotationSequenceAxes=FollowerAxes  RotationSequence=XYX  RotationSequenceAngles=[0 0 0]  RotationSequenceAnglesUnits=deg  RotationMatrix=[1 0 0; 0 1 0; 0 0 1]
  Transform1 : sm_lib/Frames and Transforms/Rigid Transform  TranslationMethod=Cartesian  TranslationStandardOffset=0  TranslationLengthUnit=cm  TranslationStandardAxis=+Z  TranslationCartesianOffset=smiData.RigidTransform(8).translation  TranslationROffset=0  TranslationROffsetUnits=m  TranslationZOffset=0  TranslationZOffsetUnits=m  TranslationThetaOffset=0  TranslationThetaOffsetUnits=deg  RotationMethod=ArbitraryAxis  RotationAngleUnits=rad  RotationStandardAxis=+Z  RotationAngle=smiData.RigidTransform(8).angle  RotationArbitraryAxis=smiData.RigidTransform(8).axis  FollAlignAxisA=+X  BaseAlignAxisA=+Y  FollAlignAxisB=+Y  BaseAlignAxisB=+Z  RotationSequenceAxes=FollowerAxes  RotationSequence=XYX  RotationSequenceAngles=[0 0 0]  RotationSequenceAnglesUnits=deg  RotationMatrix=[1 0 0; 0 1 0; 0 0 1]
  Transform2 : sm_lib/Frames and Transforms/Rigid Transform  TranslationMethod=Cartesian  TranslationStandardOffset=0  TranslationLengthUnit=cm  TranslationStandardAxis=+Z  TranslationCartesianOffset=smiData.RigidTransform(9).translation  TranslationROffset=0  TranslationROffsetUnits=m  TranslationZOffset=0  TranslationZOffsetUnits=m  TranslationThetaOffset=0  TranslationThetaOffsetUnits=deg  RotationMethod=ArbitraryAxis  RotationAngleUnits=rad  RotationStandardAxis=+Z  RotationAngle=smiData.RigidTransform(9).angle  RotationArbitraryAxis=smiData.RigidTransform(9).axis  FollAlignAxisA=+X  BaseAlignAxisA=+Y  FollAlignAxisB=+Y  BaseAlignAxisB=+Z  RotationSequenceAxes=FollowerAxes  RotationSequence=XYX  RotationSequenceAngles=[0 0 0]  RotationSequenceAnglesUnits=deg  RotationMatrix=[1 0 0; 0 1 0; 0 0 1]
  Transform3 : sm_lib/Frames and Transforms/Rigid Transform  TranslationMethod=Cartesian  TranslationStandardOffset=0  TranslationLengthUnit=cm  TranslationStandardAxis=+Z  TranslationCartesianOffset=smiData.RigidTransform(10).translation  TranslationROffset=0  TranslationROffsetUnits=m  TranslationZOffset=0  TranslationZOffsetUnits=m  TranslationThetaOffset=0  TranslationThetaOffsetUnits=deg  RotationMethod=ArbitraryAxis  RotationAngleUnits=rad  RotationStandardAxis=+Z  RotationAngle=smiData.RigidTransform(10).angle  RotationArbitraryAxis=smiData.RigidTransform(10).axis  FollAlignAxisA=+X  BaseAlignAxisA=+Y  FollAlignAxisB=+Y  BaseAlignAxisB=+Z  RotationSequenceAxes=FollowerAxes  RotationSequence=XYX  RotationSequenceAngles=[0 0 0]  RotationSequenceAnglesUnits=deg  RotationMatrix=[1 0 0; 0 1 0; 0 0 1]
  Transform4 : sm_lib/Frames and Transforms/Rigid Transform  TranslationMethod=Cartesian  TranslationStandardOffset=0  TranslationLengthUnit=cm  TranslationStandardAxis=+Z  TranslationCartesianOffset=smiData.RigidTransform(235).translation  TranslationROffset=0  TranslationROffsetUnits=m  TranslationZOffset=0  TranslationZOffsetUnits=m  TranslationThetaOffset=0  TranslationThetaOffsetUnits=deg  RotationMethod=ArbitraryAxis  RotationAngleUnits=rad  RotationStandardAxis=+Z  RotationAngle=smiData.RigidTransform(235).angle  RotationArbitraryAxis=smiData.RigidTransform(235).axis  FollAlignAxisA=+X  BaseAlignAxisA=+Y  FollAlignAxisB=+Y  BaseAlignAxisB=+Z  RotationSequenceAxes=FollowerAxes  RotationSequence=XYX  RotationSequenceAngles=[0 0 0]  RotationSequenceAnglesUnits=deg  RotationMatrix=[1 0 0; 0 1 0; 0 0 1]
  Transform5 : PMIOPort  Side=Left
  connections:
  DJI_S900_Lower_Assembly_STEP_1_RIGID/RConn1 -- Transform5/RConn1 -- Transform3/LConn1 -- Transform4/LConn1 -- Transform2/LConn1 -- Transform1/LConn1 -- Transform/LConn1
  DJI_S900_GPS_Compass_STEP_1_RIGID/LConn1 -- Transform2/RConn1
  DJI_S900_GPS_Module_STEP_1_RIGID/LConn1 -- Transform3/RConn1
  DJI_S900_A2_IMU_STEP_1_RIGID/LConn1 -- Transform1/RConn1
  DJI_S900_Landing_Bracket_Attachment_Piece_STEP_1_RIGID/LConn1 -- Transform4/RConn1
  DJI_S900_Landing_Bracket_Attachment_Piece_STEP_2_RIGID/LConn1 -- Transform/RConn1
